simulink model "microchip_mcb_pmsm_foc_qep"  (R2021b)
settings: Solver=FixedStepDiscrete  StartTime=0.0  StopTime=8  FixedStep=Ts/2  RelTol=1e-3  EnableMultiTasking=on
InitFcn:
  | microchip_mcb_pmsm_foc_qep_data
values from neighbouring files (symbols this model uses):
  inverter = mcb_SetInverterParameters('Microchip_inverter')    [microchip_mcb_pmsm_foc_qep_data.m]
  PI_params = mcb.internal.SetControllerParameters(pmsm,inverter,PU_System,T_pwm,2*Ts,Ts_speed)    [microchip_mcb_pmsm_foc_qep_data.m]
  pmsm = mcb_SetPMSMMotorParameters('Microchip_motor')    [microchip_mcb_pmsm_foc_qep_data.m]
  PU_System = mcb_SetPUSystem(pmsm,inverter)    [microchip_mcb_pmsm_foc_qep_data.m]
  PWM_frequency = 20e3    (= 20000)    [microchip_mcb_pmsm_foc_qep_data.m]
  Ts = T_pwm    (= 5e-05)    [microchip_mcb_pmsm_foc_qep_data.m]
  Ts_motor = T_pwm/2    (= 2.5e-05)    [microchip_mcb_pmsm_foc_qep_data.m]
  Ts_simulink = T_pwm/2    (= 2.5e-05)    [microchip_mcb_pmsm_foc_qep_data.m]
  Ts_speed = 10*Ts    (= 0.0005)    [microchip_mcb_pmsm_foc_qep_data.m]
undefined symbols (not defined in the file or in its folder): A24, AD10, AD7, ADC0, LQFP144, MaxPer, ms, ns, PA0, PA1, PA10, PA11, PA12, PA13, PA18, PA9, PB0, PD18, PD19, PD24, PD25, PD26, Pin, Resol, SAME70Q21B, Unsigned, Vd_Ref_openLoop_PU
libraries: mcbcontrolslib x15, MCHP_Blockset x12, simulink x11, mcbpositiondecoderlib x4, mcbplantlib x1, autolibpmsmexterior x1
(part 3 of 4)

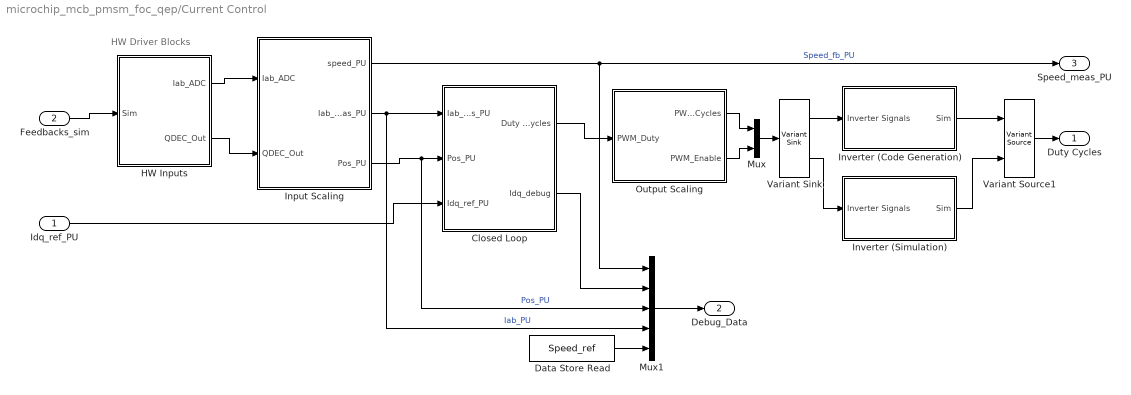
== system microchip_mcb_pmsm_foc_qep/Current Control ==
  note: HW Driver Blocks
  Idq_ref_PU : Inport
  Feedbacks_sim : Inport  Port=2
  Closed Loop : Subsystem
  Data Store Read : DataStoreRead  DataStoreName=Speed_ref  IndexOptions=Index vector (dialog)  Indices=1  OutputSizes=1
  HW Inputs : Subsystem  Variant=on  VariantControlMode=sim codegen switching
  Input Scaling : Subsystem
  Inverter (Code Generation) : Subsystem
  Inverter (Simulation) : Subsystem
  Mux : Mux  Inputs=2
  Mux1 : Mux  Inputs=5
  Output Scaling : Subsystem
  Variant Sink : VariantSink
  Variant Source1 : VariantSource
  Duty Cycles : Outport  InitialOutput=0  VectorParamsAs1DForOutWhenUnconnected=off
  Debug_Data : Outport  Port=2
  Speed_meas_PU : Outport  Port=3  InitialOutput=0  VectorParamsAs1DForOutWhenUnconnected=off
  wires:
  Closed Loop/1(Duty Cycles) -> Output Scaling/1(PWM_Duty)
  Output Scaling/2(PWM_Enable) -> Mux/2
  Input Scaling/1(speed_PU) -> Mux1/1, Speed_meas_PU/1  "Speed_fb_PU"
  Feedbacks_sim/1 -> HW Inputs/1(Sim)
  Input Scaling/2(Iab_meas_PU) -> Mux1/4, Closed Loop/1(Iab_meas_PU)  "Iab_PU"
  Input Scaling/3(Pos_PU) -> Mux1/3, Closed Loop/2(Pos_PU)  "Pos_PU"
  Variant Source1/1 -> Duty Cycles/1
  Output Scaling/1(PWM_Duty_Cycles) -> Mux/1
  Variant Sink/2 -> Inverter (Simulation)/1(Inverter Signals)
  Inverter (Code Generation)/1(Sim) -> Variant Source1/1
  Inverter (Simulation)/1(Sim) -> Variant Source1/2
  Variant Sink/1 -> Inverter (Code Generation)/1(Inverter Signals)
  Mux/1 -> Variant Sink/1
  HW Inputs/1(Iab_ADC) -> Input Scaling/1(Iab_ADC)
  HW Inputs/2(QDEC_Out) -> Input Scaling/2(QDEC_Out)
  Idq_ref_PU/1 -> Closed Loop/3(Idq_ref_PU)
  Mux1/1 -> Debug_Data/1
  Closed Loop/2(Idq_debug) -> Mux1/2
  Data Store Read/1 -> Mux1/5

== system microchip_mcb_pmsm_foc_qep/Heartbeat LED ==
  note: Heartbeat LED 1HZ
  Code generation : Subsystem
  RED_LED : Constant  OutDataTypeStr=uint16  SampleTime=0.25
  Simulation : Subsystem
  Variant Sink : VariantSink
  wires:
  RED_LED/1 -> Variant Sink/1
  Variant Sink/1 -> Code generation/1(In1)
  Variant Sink/2 -> Simulation/1(In1)

== system microchip_mcb_pmsm_foc_qep/Inverter and Motor - Plant Model ==
  Duty_Cycles : Inport
  Plant Model : Subsystem  Variant=on  VariantControlMode=sim codegen switching  VariantControl=Variant1  PropagateVariantConditions=on
  Feedbacks_sim : Outport  VectorParamsAs1DForOutWhenUnconnected=off
  wires:
  Duty_Cycles/1 -> Plant Model/1(Duty_Cycles)
  Plant Model/1(Feedbacks_sim) -> Feedbacks_sim/1

== system microchip_mcb_pmsm_foc_qep/Serial Receive ==
  CodeGen : Subsystem
  Data Store Write : DataStoreWrite  DataStoreName=Enable  IndexOptions=Index vector (dialog)  Indices=1  OutputSizes=1
  Sim : Subsystem
  Variant Source : VariantSource  VariantControlMode=sim codegen switching
  Variant Source1 : VariantSource  VariantControlMode=sim codegen switching
  SpeedRef : Outport
  wires:
  Variant Source/1 -> SpeedRef/1
  Variant Source1/1 -> Data Store Write/1
  Sim/1(SpeedRef) -> Variant Source/2
  Sim/2(Enable) -> Variant Source1/2
  CodeGen/1(SpeedRef) -> Variant Source/1
  CodeGen/2(Enable) -> Variant Source1/1

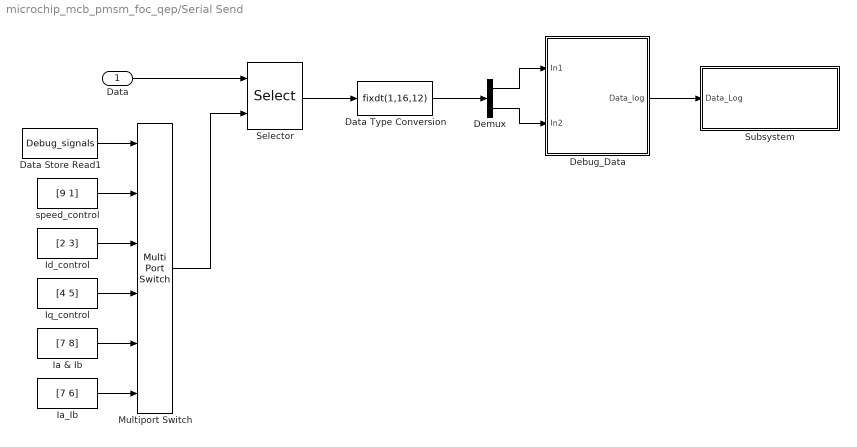
== system microchip_mcb_pmsm_foc_qep/Serial Send ==
  Data : Inport
  Data Store Read1 : DataStoreRead  DataStoreName=Debug_signals  IndexOptions=Index vector (dialog)  Indices=1  OutputSizes=1
  Data Type Conversion : DataTypeConversion  OutDataTypeStr=fixdt(1,16,12)  RndMeth=Simplest
  Debug_Data : Subsystem
  Demux : Demux  Outputs=2
  Ia & Ib : Constant  Value=[7 8]  OutDataTypeStr=uint16  SampleTime=-1
  Ia_Ib : Constant  Value=[7 6]  OutDataTypeStr=uint16  SampleTime=-1
  Id_control : Constant  Value=[2 3]  OutDataTypeStr=uint16  SampleTime=-1
  Iq_control : Constant  Value=[4 5]  OutDataTypeStr=uint16  SampleTime=-1
  Multiport Switch : MultiPortSwitch  Inputs=5  DiagnosticForDefault=Warning  OutDataTypeStr=uint16  RndMeth=Simplest
  Selector : Selector  InputPortWidth=9  IndexOptions=Index vector (port)  Indices=[1 3]  OutputSizes=1
  Subsystem : Subsystem
  speed_control : Constant  Value=[9 1]  OutDataTypeStr=uint16  SampleTime=-1
  wires:
  Debug_Data/1(Data_log) -> Subsystem/1(Data_Log)
  Demux/1 -> Debug_Data/1(In1)
  Demux/2 -> Debug_Data/2(In2)
  Data Type Conversion/1 -> Demux/1
  Selector/1 -> Data Type Conversion/1
  Data/1 -> Selector/1
  Data Store Read1/1 -> Multiport Switch/1
  Multiport Switch/1 -> Selector/2
  Ia_Ib/1 -> Multiport Switch/6
  Ia & Ib/1 -> Multiport Switch/5
  Iq_control/1 -> Multiport Switch/4
  Id_control/1 -> Multiport Switch/3
  speed_control/1 -> Multiport Switch/2

== system microchip_mcb_pmsm_foc_qep/Speed Control ==
  In1 : Inport
  Speed_Meas_PU : Inport  Port=2
  Data Store Write3 : DataStoreWrite  DataStoreName=Speed_ref  IndexOptions=Index vector (dialog)  Indices=1  OutputSizes=1
  Id_Ref : Constant  Value=0  OutDataTypeStr=dataType
  Mux : Mux  Inputs=2
  PI_Controller_Speed : Subsystem
  Speed_Ref_Selector : Subsystem
  IdqRef_PU : Outport  VectorParamsAs1DForOutWhenUnconnected=off
  wires:
  PI_Controller_Speed/1(Iq_ref) -> Mux/2
  Speed_Meas_PU/1 -> PI_Controller_Speed/2(N_fb)  "Speed_fb"
  Id_Ref/1 -> Mux/1
  Mux/1 -> IdqRef_PU/1
  Speed_Ref_Selector/1(Speed_Ref1) -> PI_Controller_Speed/1(N_ref)  "Speed_ref"
  In1/1 -> Data Store Write3/1, Speed_Ref_Selector/1(Speed_Ref)

== system microchip_mcb_pmsm_foc_qep/Current Control/Closed Loop ==
  Iab_meas_PU : Inport
  Pos_PU : Inport  Port=2
  Idq_ref_PU : Inport  Port=3
  Data Store Read1 : DataStoreRead  DataStoreName=EnClosedLoop  IndexOptions=Index vector (dialog)  Indices=1  OutputSizes=1
  Merge : Merge
  NOT : Logic  Operator=NOT  IconShape=distinctive  AllPortsSameDT=off  OutDataTypeStr=boolean
  OpenLoop : Subsystem
  Subsystem : Subsystem
  Duty Cycles : Outport  VectorParamsAs1DForOutWhenUnconnected=off
  Idq_debug : Outport  Port=2  VectorParamsAs1DForOutWhenUnconnected=off
  wires:
  Iab_meas_PU/1 -> Subsystem/1(Iab_meas_PU)  "Ia_Ib"
  Pos_PU/1 -> Subsystem/2(Pos_PU)
  Idq_ref_PU/1 -> Subsystem/3(Idq_ref_PU)
  Subsystem/1(Idq_debug) -> Idq_debug/1
  Merge/1 -> Duty Cycles/1
  OpenLoop/1(Duty Cycles) -> Merge/2
  Subsystem/2(Duty Cycles) -> Merge/1
  Data Store Read1/1 -> NOT/1, Subsystem/Enable
  NOT/1 -> OpenLoop/Enable

== system microchip_mcb_pmsm_foc_qep/Current Control/HW Inputs ==
  Sim : Inport
  Sensor Driver Blocks (codegen) : Subsystem  VariantControl=(codegen)
  Sensor Driver Blocks (sim) : Subsystem  VariantControl=(sim)
  Iab_ADC : Outport
  QDEC_Out : Outport  Port=2

== system microchip_mcb_pmsm_foc_qep/Current Control/Input Scaling ==
  Iab_ADC : Inport
  QDEC_Out : Inport  Port=2
  Calculate Phase Currents : Subsystem
  Calculate Position and Speed : Subsystem
  speed_PU : Outport
  Iab_meas_PU : Outport  Port=2
  Pos_PU : Outport  Port=3
  wires:
  Calculate Phase Currents/1(Iab_meas_PU) -> Iab_meas_PU/1
  Iab_ADC/1 -> Calculate Phase Currents/1(Iab_ADC)
  QDEC_Out/1 -> Calculate Position and Speed/1(Count)
  Calculate Position and Speed/1(Out1) -> speed_PU/1
  Calculate Position and Speed/2(ϴe) -> Pos_PU/1

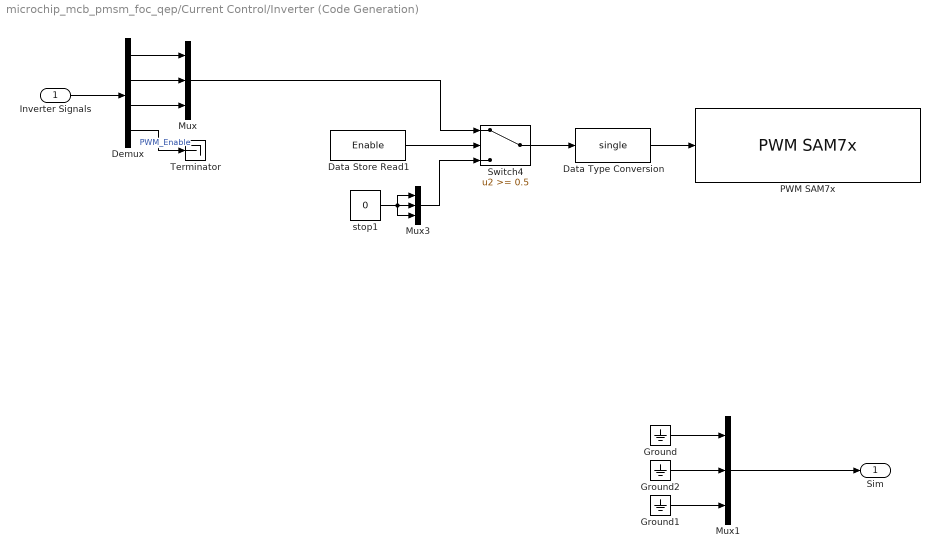
== system microchip_mcb_pmsm_foc_qep/Current Control/Inverter (Code Generation) ==
  Inverter Signals : Inport
  Data Store Read1 : DataStoreRead  DataStoreName=Enable  IndexOptions=Index vector (dialog)  Indices=1  OutputSizes=1
  Data Type Conversion : DataTypeConversion  OutDataTypeStr=single
  Demux : Demux
  Ground : Ground
  Ground1 : Ground
  Ground2 : Ground
  Mux : Mux  Inputs=3
  Mux1 : Mux  Inputs=3
  Mux3 : Mux  Inputs=3
  PWM SAM7x : MCHP_Blockset/PWM IO/PWM SAM7x  Priority=-2000  PWMx=PWM Controller 0  MaxPeriod_s=50e-6  PWM0_pinH0=Dynamic Options  PWM0_pinH0_TXT=PA11 / Pin[64]  PWM0_pinL0=Dynamic Options  PWM0_pinL0_TXT=PD24 / Pin[55]  PWM0_pinH1=Dynamic Options  PWM0_pinH1_TXT=PA12 / Pin[68]  PWM0_pinL1=Dynamic Options  PWM0_pinL1_TXT=PD25 / Pin[52]  PWM0_pinH2=Dynamic Options  PWM0_pinH2_TXT=PA13 / Pin[42]  PWM0_pinL2=Dynamic Options  PWM0_pinL2_TXT=PD26 / Pin[53]  PWM0_pinH3=Dynamic Options  PWM0_pinH3_TXT=Not Used  PWM0_pinL3=Dynamic Options  PWM0_pinL3_TXT=Not Used  PWM1_pinH0=Dynamic Options  PWM1_pinH0_TXT=Not Used  PWM1_pinL0=Dynamic Options  PWM1_pinL0_TXT=Not Used  PWM1_pinH1=Dynamic Options  PWM1_pinH1_TXT=Not Used  PWM1_pinL1=Dynamic Options  PWM1_pinL1_TXT=Not Used  PWM1_pinH2=Dynamic Options  PWM1_pinH2_TXT=Not Used  PWM1_pinL2=Dynamic Options  PWM1_pinL2_TXT=Not Used  PWM1_pinH3=Dynamic Options  PWM1_pinH3_TXT=Not Used  PWM1_pinL3=Dynamic Options  PWM1_pinL3_TXT=Not Used  PWM_Centered=on  PWM_SyncWithPWM0=on  PushPull_Mode=off  SampleTime=Ts  S_INPUT=[-1]  S_INPUT_Size=[3]  S_OUTPUT=[]  S_OUTPUT_Size=[]  S_ListCustomDatatype=S.S_ListCustomDatatype={};  evalin_ws=PWM0max0=MCHP_Fun.Hex2num('40AD4C0000000000');PWM1max0=MCHP_Fun.Hex2num('40AD4C0000000000');PWM2max0=MCHP_Fun.Hex2num('40AD4C0000000000');  MCHP_PWMC_CLOCK_REQUEST=''  MCHP_PWMC_CLOCK_RESULT=''  MCHP_USER_INTERRUPTS=0  MCHP_PORT={PWM0H0 }{PWMH0}4:1:P11;{PWM0L0 }{PWML0}4:1:P120;{PWM0H1 }{PWMH1}4:1:P12;{PWM0L1 }{PWML1}4:1:P121;{PWM0H2 }{PWMH2}4:1:P13;{PWM0L2 }{PWML2}4:1:P122;  MCHP_MASTERLINK=microchip_mcb_pmsm_foc_qep/Configurations/Microchip Master  invert_PWMH0=off  invert_PWML0=off  invert_PWMH1=off  invert_PWML1=off  invert_PWMH2=off  invert_PWML2=off  invert_PWMH3=off  invert_PWML3=off  InitPeriod_s=50e-6  InitDutyCycle_s=0  InitDeadTimeH_s=1e-6  InitDeadTimeL_s=1e-6  InitEventLine0_ComparatorValue_s=1e-7  InitEventLine1_ComparatorValue_s=[]  BlockInput_VectorScalar=Vectors (grouped by function)  BlockInput_Period=Not a block input  BlockInput_DutyCycle=a Floating Point input within range [-1 1]  BlockInput_DeadTime=Not a block input  BlockInput_OutputOverride=Not a block input  Fault_FPV0=Not forced  Fault_FPV1=Not forced  Fault_FPV2=Not forced  Fault_FPV3=Not forced  Fault_Input0=does nothing  Fault_Input0_FFIL=off  Fault_Input1=does nothing  Fault_Input1_FFIL=off  Fault_Input2=does nothing  Fault_Input2_FFIL=on  Fault_Input3=does nothing  Fault_Input3_FFIL=off  Fault_Input4=does nothing  Fault_Input4_FFIL=on  Fault_Input5=does nothing  Fault_Input5_FFIL=on  Fault_Input6=does nothing  Fault_Input6_FFIL=on  Fault_Input7=does nothing  Fault_Input7_FFIL=on
      settings: SourceProductName=MPLAB Device Blocks for Simulink
  Switch4 : Switch  Threshold=0.5  RndMeth=Simplest
  Terminator : Terminator
  stop1 : Constant  Value=0  OutDataTypeStr=dataType
  Sim : Outport  VectorParamsAs1DForOutWhenUnconnected=off
  wires:
  Inverter Signals/1 -> Demux/1
  Ground/1 -> Mux1/1
  Ground1/1 -> Mux1/3
  Ground2/1 -> Mux1/2
  Mux1/1 -> Sim/1
  Demux/1 -> Mux/1
  Demux/2 -> Mux/2
  Demux/3 -> Mux/3
  Switch4/1 -> Data Type Conversion/1
  Data Store Read1/1 -> Switch4/2
  Data Type Conversion/1 -> PWM SAM7x/1
  stop1/1 -> Mux3/3, Mux3/2, Mux3/1
  Mux/1 -> Switch4/1
  Mux3/1 -> Switch4/3
  Demux/4 -> Terminator/1  "PWM_Enable"

== system microchip_mcb_pmsm_foc_qep/Current Control/Inverter (Simulation) ==
  Inverter Signals : Inport
  Data Type Duplicate : DataTypeDuplicate
  Demux : Demux
  Mux : Mux  Inputs=3
  Mux2 : Mux  Inputs=3
  Subsystem : Subsystem
  Switch1 : Switch  Threshold=0.5  RndMeth=Simplest
  stop : Constant  Value=0  OutDataTypeStr=Inherit: Inherit via back propagation
  Sim : Outport  VectorParamsAs1DForOutWhenUnconnected=off
  wires:
  stop/1 -> Data Type Duplicate/2, Mux2/1, Mux2/3, Mux2/2
  Mux2/1 -> Switch1/3
  Switch1/1 -> Sim/1
  Inverter Signals/1 -> Demux/1
  Demux/4 -> Switch1/2  "PWM Enable"
  Mux/1 -> Subsystem/1(In1), Data Type Duplicate/1  "PWM Duty Cycles"
  Demux/1 -> Mux/1
  Demux/2 -> Mux/2
  Demux/3 -> Mux/3
  Subsystem/1(PWM_Duty_Cycles) -> Switch1/1  "test"

== system microchip_mcb_pmsm_foc_qep/Current Control/Output Scaling ==
  PWM_Duty : Inport
  Data Type Conversion : DataTypeConversion  OutDataTypeStr=dataType
  Enable : DataStoreRead  DataStoreName=Enable  IndexOptions=Index vector (dialog)  Indices=1  OutputSizes=1
  PWM_Duty_Cycles : Outport
  PWM_Enable : Outport  Port=2
  wires:
  Data Type Conversion/1 -> PWM_Enable/1
  Enable/1 -> Data Type Conversion/1
  PWM_Duty/1 -> PWM_Duty_Cycles/1

== system microchip_mcb_pmsm_foc_qep/Heartbeat LED/Code generation ==
  In1 : Inport
  DBG LED 1 : MCHP_Blockset/Digital IO/Digital Output Write  PORT=Dynamic Options  PORT_TXT="C   [ 0 : 31 ]"  PIN=23  PACK=off  SIMULTANEOUS=off  ORDERING=None  SampleTime=-1  MCHP_PORT={Digital Out}{DOU}1:1:C23;  MCHP_MASTERLINK=microchip_mcb_pmsm_foc_qep/Configurations/Microchip Master
      settings: SourceProductName=MPLAB Device Blocks for Simulink
  Delay 10Hz : Delay  DelayLength=1  InitialCondition=0  SampleTime=0.25
  Logical Operator : Logic  Operator=NOT  AllPortsSameDT=off  OutDataTypeStr=boolean
  Terminator : Terminator
  wires:
  Logical Operator/1 -> DBG LED 1/1, Delay 10Hz/1
  Delay 10Hz/1 -> Logical Operator/1
  In1/1 -> Terminator/1

== system microchip_mcb_pmsm_foc_qep/Heartbeat LED/Simulation ==
  In1 : Inport
  Simulation_Terminator : Terminator
  wires:
  In1/1 -> Simulation_Terminator/1

== system microchip_mcb_pmsm_foc_qep/Inverter and Motor - Plant Model/Plant Model ==
  Duty_Cycles : Inport
  Inverter and Motor (codegen) : Subsystem  VariantControl=(codegen)
  Inverter and Motor (sim) : Subsystem  VariantControl=(sim)
  Feedbacks_sim : Outport  VectorParamsAs1DForOutWhenUnconnected=off

== system microchip_mcb_pmsm_foc_qep/Serial Receive/CodeGen ==
  Data Store Write1 : DataStoreWrite  DataStoreName=Debug_signals  IndexOptions=Index vector (dialog)  Indices=1  OutputSizes=1
  Data Type Conversion : DataTypeConversion  OutDataTypeStr=uint16
  Subsystem : Subsystem
  Subsystem1 : Subsystem
  UART Rx : MCHP_Blockset/BUS UART/UART Rx  UART_REF=UART 0  Flag_Out=on  Rx_Size_popup=User defined  Rx_Size=1  S_Rx_Size=1  Split=Read all received char  SplitChar=10  OutputDefault_popup=do nothing (end of output vector will be undefined)  OutputDefault=-2  ORDERING=None  SampleTime=.001  MCHP_MASTERLINK=microchip_mcb_pmsm_foc_qep/Configurations/Microchip Master  MCHP_COMPILED_INFO="CompiledSampleTime= [0.0010000000000000000208   0 ];CompiledInportDataTypes=[    ];CompiledInportDataWidth=[];"
      settings: SourceProductName=MPLAB Device Blocks for Simulink
  SpeedRef : Outport
  Enable : Outport  Port=2
  wires:
  UART Rx/1 -> Data Type Conversion/1
  Subsystem/3(Debug Signal Selection) -> Data Store Write1/1
  UART Rx/2 -> Subsystem1/1(In1)
  Subsystem/2(Enable) -> Enable/1
  Subsystem/1(SpeedRef) -> SpeedRef/1
  Subsystem1/2(Data out) -> Subsystem/1(In1)
  Subsystem1/1(NewData) -> Subsystem/Enable
  Data Type Conversion/1 -> Subsystem1/Enable

== system microchip_mcb_pmsm_foc_qep/Serial Receive/Sim ==
  Data Type Conversion1 : DataTypeConversion  OutDataTypeStr=dataType  RndMeth=Simplest
  Data Type Conversion2 : DataTypeConversion  OutDataTypeStr=boolean  RndMeth=Simplest
  Step : Step  Time=5  Before=0.5  After=-0.5  OutDataTypeStr=single  SampleTime=0.001
  Step1 : Step  OutDataTypeStr=single  SampleTime=0.001
  SpeedRef : Outport
  Enable : Outport  Port=2
  wires:
  Step/1 -> Data Type Conversion1/1
  Data Type Conversion1/1 -> SpeedRef/1
  Step1/1 -> Data Type Conversion2/1
  Data Type Conversion2/1 -> Enable/1

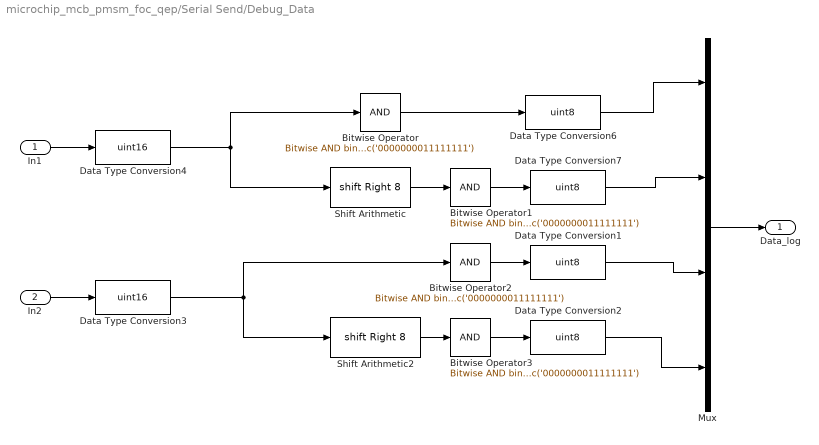
== system microchip_mcb_pmsm_foc_qep/Serial Send/Debug_Data ==
  In1 : Inport
  In2 : Inport  Port=2
  Bitwise Operator{,1..3} (4 alike) : simulink/Logic and Bit Operations/Bitwise Operator  logicop=AND  UseBitMask=on  BitMask=bin2dec('0000000011111111')  BitMaskRealWorld=Stored Integer
  Data Type Conversion{1..2,6..7} (4 alike) : DataTypeConversion  OutDataTypeStr=uint8  RndMeth=Simplest
  Data Type Conversion3 : DataTypeConversion  OutDataTypeStr=uint16  ConvertRealWorld=Stored Integer (SI)  RndMeth=Simplest
  Data Type Conversion4 : DataTypeConversion  OutDataTypeStr=uint16  ConvertRealWorld=Stored Integer (SI)  RndMeth=Simplest
  Mux : Mux
  Shift Arithmetic : ArithShift  BitShiftNumber=8  BitShiftDirection=Right
  Shift Arithmetic2 : ArithShift  BitShiftNumber=8  BitShiftDirection=Right
  Data_log : Outport
  wires:
  Data Type Conversion3/1 -> Bitwise Operator2/1, Shift Arithmetic2/1
  Bitwise Operator3/1 -> Data Type Conversion2/1
  Shift Arithmetic2/1 -> Bitwise Operator3/1
  Bitwise Operator1/1 -> Data Type Conversion7/1
  Data Type Conversion2/1 -> Mux/4
  Shift Arithmetic/1 -> Bitwise Operator1/1
  Bitwise Operator/1 -> Data Type Conversion6/1
  Data Type Conversion1/1 -> Mux/3
  Bitwise Operator2/1 -> Data Type Conversion1/1
  Data Type Conversion7/1 -> Mux/2
  Data Type Conversion6/1 -> Mux/1
  Data Type Conversion4/1 -> Shift Arithmetic/1, Bitwise Operator/1
  In1/1 -> Data Type Conversion4/1
  In2/1 -> Data Type Conversion3/1
  Mux/1 -> Data_log/1

== system microchip_mcb_pmsm_foc_qep/Serial Send/Subsystem ==
  note: Fast Serial Data Monitoring (32-bit)
  Data_Log : Inport
  Counter Limited : simulink/Sources/Counter Limited  uplimit=119  tsamp=-1
  Data : Subsystem  TreatAsAtomicUnit=on
  End : Subsystem  TreatAsAtomicUnit=on
  If : If  IfExpression=u1 == 0  ElseIfExpressions=u1 == 119
  Start : Subsystem  TreatAsAtomicUnit=on
  wires:
  If/3 -> Data/Action
  Counter Limited/1 -> If/1
  If/2 -> End/Action
  If/1 -> Start/Action
  Data_Log/1 -> End/1(Data), Start/1(Data), Data/1(Data)

== system microchip_mcb_pmsm_foc_qep/Speed Control/PI_Controller_Speed ==
  N_ref : Inport
  N_fb : Inport  Port=2
  AND : Logic  IconShape=distinctive  AllPortsSameDT=off  OutDataTypeStr=boolean
  Data Store Read2 : DataStoreRead  DataStoreName=EnClosedLoop  IndexOptions=Index vector (dialog)  Indices=1  OutputSizes=1
  Data Store Read1 : DataStoreRead  DataStoreName=Enable  IndexOptions=Index vector (dialog)  Indices=1  OutputSizes=1
  Discrete PI Controller with anti-windup & reset : mcbcontrolslib/Discrete PI Controller  with anti-windup & reset  UpperSaturationLimit=0.5  LowerSaturationLimit=-0.5
      settings: SourceProductBaseCode=MT
  Ki1 : Constant  Value=PI_params.Ki_speed*Ts_speed  OutDataTypeStr=dataType  SampleTime=-1
  Ki2 : Constant  Value=0  OutDataTypeStr=dataType  SampleTime=-1
  Kp1 : Constant  Value=PI_params.Kp_speed  OutDataTypeStr=dataType  SampleTime=-1
  Logical Operator : Logic  Operator=NOT  IconShape=distinctive  AllPortsSameDT=off  OutDataTypeStr=boolean
  Sum : Sum  Inputs=|+-  OutDataTypeStr=Inherit: Same as first input
  Iq_ref : Outport  VectorParamsAs1DForOutWhenUnconnected=off
  wires:
  Discrete PI Controller with anti-windup & reset/1 -> Iq_ref/1
  Ki1/1 -> Discrete PI Controller with anti-windup & reset/3
  Kp1/1 -> Discrete PI Controller with anti-windup & reset/2
  N_fb/1 -> Sum/2
  N_ref/1 -> Sum/1
  Sum/1 -> Discrete PI Controller with anti-windup & reset/1
  Logical Operator/1 -> Discrete PI Controller with anti-windup & reset/4
  Ki2/1 -> Discrete PI Controller with anti-windup & reset/5
  Data Store Read1/1 -> AND/1
  Data Store Read2/1 -> AND/2
  AND/1 -> Logical Operator/1

== system microchip_mcb_pmsm_foc_qep/Speed Control/Speed_Ref_Selector ==
  Speed_Ref : Inport
  Constant : Constant  Value=0  OutDataTypeStr=dataType
  Constant1 : Constant  Value=-0.1  OutDataTypeStr=dataType
  Data Store Read : DataStoreRead  DataStoreName=Speed_ref  IndexOptions=Index vector (dialog)  Indices=1  OutputSizes=1
  Data Store Read1 : DataStoreRead  DataStoreName=EnClosedLoop  IndexOptions=Index vector (dialog)  Indices=1  OutputSizes=1
  IIR Filter : mcbcontrolslib/IIR Filter  VariantControl=Low Pass Filter  VariantSelect=Low-pass  Filter_constant=0.001*(Ts_speed/Ts)  advancedSettings=off  Ts=50e-6  cutOff_freq=32.1525
      settings: SourceProductBaseCode=MT
  Switch : Switch  Criteria=u2 > Threshold
  Switch1 : Switch  Criteria=u2 > Threshold
  Speed_Ref1 : Outport
  wires:
  IIR Filter/1 -> Speed_Ref1/1  "Speed_Ref"
  Data Store Read1/1 -> Switch/2
  Switch/1 -> IIR Filter/1  "Speed_Ref"
  Constant/1 -> Switch1/1
  Data Store Read/1 -> Switch1/2
  Switch1/1 -> Switch/3
  Speed_Ref/1 -> Switch/1
  Constant1/1 -> Switch1/3

== system microchip_mcb_pmsm_foc_qep/Current Control/Closed Loop/OpenLoop ==
  Enable : EnablePort
  Constant : Constant  Value=0.15  OutDataTypeStr=dataType
  Constant1 : Constant  Value=0  OutDataTypeStr=dataType
  Enable1 : DataStoreRead  DataStoreName=Enable  IndexOptions=Index vector (dialog)  Indices=1  OutputSizes=1
  Inverse Park Transform : mcbcontrolslib/Inverse Park Transform  AxisAlignment=D-axis
  Mode Selector : Subsystem
  Mux1 : Mux  Inputs=3
  Sine-Cosine Lookup : mcbcontrolslib/Sine-Cosine Lookup  AngleInput=Per-unit  N_points=1024
      settings: SourceProductBaseCode=MT
  Space Vector Generator : mcbcontrolslib/PWM Reference Generator  inSignal=Valphabeta  modType=SVM: space vector modulation
      settings: SourceProductBaseCode=MT
  Duty Cycles : Outport  VectorParamsAs1DForOutWhenUnconnected=off
  wires:
  Mode Selector/1(PositionOffsetEn) -> Sine-Cosine Lookup/1  "Pos_open"
  Constant1/1 -> Inverse Park Transform/2
  Constant/1 -> Inverse Park Transform/1
  Space Vector Generator/3 -> Mux1/3
  Sine-Cosine Lookup/2 -> Inverse Park Transform/4
  Space Vector Generator/1 -> Mux1/1
  Sine-Cosine Lookup/1 -> Inverse Park Transform/3
  Inverse Park Transform/2 -> Space Vector Generator/2
  Space Vector Generator/2 -> Mux1/2
  Inverse Park Transform/1 -> Space Vector Generator/1
  Mux1/1 -> Duty Cycles/1
  Enable1/1 -> Mode Selector/Enable

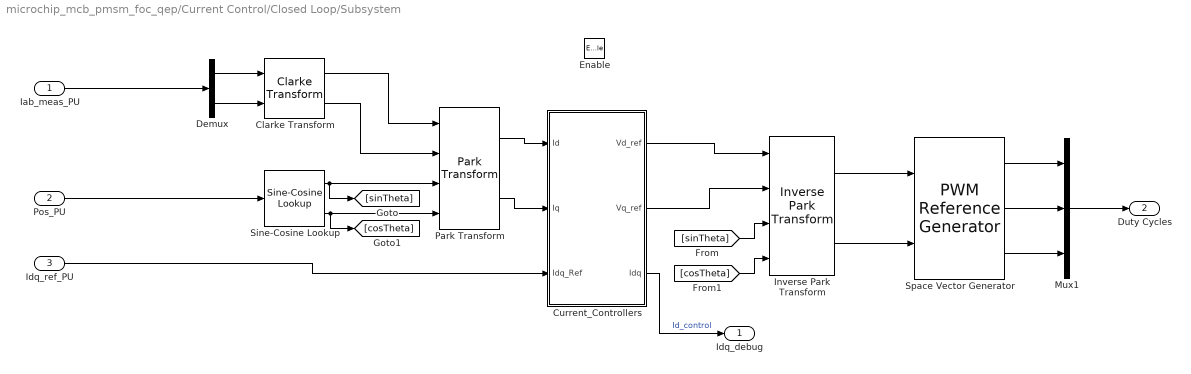
== system microchip_mcb_pmsm_foc_qep/Current Control/Closed Loop/Subsystem ==
  Iab_meas_PU : Inport
  Pos_PU : Inport  Port=2
  Idq_ref_PU : Inport  Port=3
  Enable : EnablePort
  Clarke Transform : mcbcontrolslib/Clarke Transform  VariantControl=Variant2
  Current_Controllers : Subsystem
  Demux : Demux  Outputs=2
  Inverse Park Transform : mcbcontrolslib/Inverse Park Transform  AxisAlignment=D-axis
  Mux1 : Mux  Inputs=3
  Park Transform : mcbcontrolslib/Park Transform  AxisAlignment=D-axis
      settings: SourceProductBaseCode=MT
  Sine-Cosine Lookup : mcbcontrolslib/Sine-Cosine Lookup  AngleInput=Per-unit  N_points=1024
      settings: SourceProductBaseCode=MT
  Space Vector Generator : mcbcontrolslib/PWM Reference Generator  inSignal=Valphabeta  modType=SVM: space vector modulation
      settings: SourceProductBaseCode=MT
  Idq_debug : Outport  VectorParamsAs1DForOutWhenUnconnected=off
  Duty Cycles : Outport  Port=2  VectorParamsAs1DForOutWhenUnconnected=off
  wires:
  Pos_PU/1 -> Sine-Cosine Lookup/1
  Inverse Park Transform/2 -> Space Vector Generator/2
  [cosTheta] -> Inverse Park Transform/4
  Inverse Park Transform/1 -> Space Vector Generator/1
  Sine-Cosine Lookup/1 -> [sinTheta], Park Transform/3
  Current_Controllers/1(Vd_ref) -> Inverse Park Transform/1
  Sine-Cosine Lookup/2 -> Park Transform/4, [cosTheta]
  Clarke Transform/2 -> Park Transform/2
  Clarke Transform/1 -> Park Transform/1
  Space Vector Generator/3 -> Mux1/3
  Space Vector Generator/1 -> Mux1/1
  Current_Controllers/3(Idq) -> Idq_debug/1  "Id_control"
  Mux1/1 -> Duty Cycles/1
  Space Vector Generator/2 -> Mux1/2
  Iab_meas_PU/1 -> Demux/1
  Demux/2 -> Clarke Transform/2
  [sinTheta] -> Inverse Park Transform/3
  Demux/1 -> Clarke Transform/1
  Park Transform/2 -> Current_Controllers/2(Iq)
  Current_Controllers/2(Vq_ref) -> Inverse Park Transform/2
  Idq_ref_PU/1 -> Current_Controllers/3(Idq_Ref)
  Park Transform/1 -> Current_Controllers/1(Id)

== system microchip_mcb_pmsm_foc_qep/Current Control/HW Inputs/Sensor Driver Blocks (codegen) ==
  Sim : Inport
  ADC SAMx1 : MCHP_Blockset/Analog IO/ADC SAMx7  Priority=-2000  AFECx=AFE Controller 0  SIGNMODE_SingleEnded=Unsigned (uint16)  SIGNMODE_Differential=Unsigned (uint16)  AFEC0_seq0=Dynamic Options  AFEC0_seq0_TXT="AD0 / PD30   &   AD6 / PA17"  AFEC1_seq0=Dynamic Options  AFEC1_seq0_TXT=Not used  AFEC0_seq1=Dynamic Options  AFEC0_seq1_TXT=AD7 / PA18  AFEC1_seq1=Dynamic Options  AFEC1_seq1_TXT=Not used  AFEC0_seq2=Dynamic Options  AFEC0_seq2_TXT=AD10 / PB0  AFEC1_seq2=Dynamic Options  AFEC1_seq2_TXT=Not used  AFEC0_seq3=Dynamic Options  AFEC0_seq3_TXT=Not used  AFEC1_seq3=Dynamic Options  AFEC1_seq3_TXT=Not used  AFEC0_seq4=Dynamic Options  AFEC0_seq4_TXT=Not used  AFEC1_seq4=Dynamic Options  AFEC1_seq4_TXT=Not used  AFEC0_seq5=Dynamic Options  AFEC0_seq5_TXT=Not used  AFEC1_seq5=Dynamic Options  AFEC1_seq5_TXT=Not used  AFEC0_seq6=Dynamic Options  AFEC0_seq6_TXT=Not used  AFEC1_seq6=Dynamic Options  AFEC1_seq6_TXT=Not used  AFEC0_seq7=Dynamic Options  AFEC0_seq7_TXT=Not used  AFEC1_seq7=Dynamic Options  AFEC1_seq7_TXT=Not used  AFEC0_seq8=Dynamic Options  AFEC0_seq8_TXT=Not used  AFEC1_seq8=Dynamic Options  AFEC1_seq8_TXT=Not used  AFEC0_seq9=Dynamic Options  AFEC0_seq9_TXT=Not used  AFEC1_seq9=Dynamic Options  AFEC1_seq9_TXT=Not used  AFEC0_seq10=Dynamic Options  AFEC0_seq10_TXT=Not used  AFEC1_seq10=Dynamic Options  AFEC1_seq10_TXT=Not used  AFEC0_seq11=Dynamic Options  AFEC0_seq11_TXT=Not used  AFEC1_seq11=Dynamic Options  AFEC1_seq11_TXT=Not used  SampleTime=Ts  S_INPUT=[-1]  S_INPUT_Size=[3]  S_OUTPUT=[]  S_OUTPUT_Size=[]  S_ListCustomDatatype=S.S_ListCustomDatatype={};  MCHP_AFECC_CLOCK_REQUEST=''  MCHP_AFECC_CLOCK_RESULT=''  MCHP_USER_INTERRUPTS=0  MCHP_PORT={AD0 AFEC0}{AD0}15:2:P126;{AD6 AFEC0}{AD6}15:2:P17;{AD7 AFEC0}{AD7}15:2:P18;{AD10 AFEC0}{AD10}15:2:P32;  MCHP_MASTERLINK=microchip_mcb_pmsm_foc_qep/Configurations/Microchip Master  Rin=< 200 Ohm  RES=12-bit Standard  AFEC0_Synchronisation=Triggered by user defined source  AFEC0_Trig=PWM0 event line 0  AFEC0_TrigTimeStep=on  AFEC1_Synchronisation=Triggered by user defined source  AFEC1_Trig=PWM1 event line 0  AFEC1_TrigTimeStep=off  ADC_TrigInfo=0  AFEC0_seq0_GAIN=1  AFEC1_seq0_GAIN=1  AFEC0_seq1_GAIN=1  AFEC1_seq1_GAIN=1  AFEC0_seq2_GAIN=1  AFEC1_seq2_GAIN=1  AFEC0_seq3_GAIN=1  AFEC1_seq3_GAIN=1  AFEC0_seq4_GAIN=1  AFEC1_seq4_GAIN=1  AFEC0_seq5_GAIN=1  AFEC1_seq5_GAIN=1  AFEC0_seq6_GAIN=1  AFEC1_seq6_GAIN=1  AFEC0_seq7_GAIN=1  AFEC1_seq7_GAIN=1  AFEC0_seq8_GAIN=1  AFEC1_seq8_GAIN=1  AFEC0_seq9_GAIN=1  AFEC1_seq9_GAIN=1  AFEC0_seq10_GAIN=1  AFEC1_seq10_GAIN=1  AFEC0_seq11_GAIN=1  AFEC1_seq11_GAIN=1  AFEC0_seq0_OFFSET=0  AFEC1_seq0_OFFSET=0  AFEC0_seq1_OFFSET=0  AFEC1_seq1_OFFSET=0  AFEC0_seq2_OFFSET=0  AFEC1_seq2_OFFSET=0  AFEC0_seq3_OFFSET=0  AFEC1_seq3_OFFSET=0  AFEC0_seq4_OFFSET=0  AFEC1_seq4_OFFSET=0  AFEC0_seq5_OFFSET=0  AFEC1_seq5_OFFSET=0  AFEC0_seq6_OFFSET=0  AFEC1_seq6_OFFSET=0  AFEC0_seq7_OFFSET=0  AFEC1_seq7_OFFSET=0  AFEC0_seq8_OFFSET=0  AFEC1_seq8_OFFSET=0  AFEC0_seq9_OFFSET=0  AFEC1_seq9_OFFSET=0  AFEC0_seq10_OFFSET=0  AFEC1_seq10_OFFSET=0  AFEC0_seq11_OFFSET=0  AFEC1_seq11_OFFSET=0
      settings: SourceProductName=MPLAB Device Blocks for Simulink
  Data Store Read : DataStoreRead  DataStoreName=EnPosOffset  IndexOptions=Index vector (dialog)  Indices=1  OutputSizes=1
  Mux : Mux  Inputs=2
  QDEC : MCHP_Blockset/QEI/QDEC  QDEC_REF=Dynamic Options  QDEC_REF_TXT=TC0  PHA_PIN=Dynamic Options  PHA_PIN_TXT=PA0 / Pin[102]  PHB_PIN=Dynamic Options  PHB_PIN_TXT=PA1 / Pin[99]  IDX_PIN=Dynamic Options  IDX_PIN_TXT=not used  INVERT_PHA=off  INVERT_PHB=off  INVERT_IDX=off  SWAP_PHA_PHB=off  SampleTime=Ts  MCHP_PORT={TC0}{TIOA0}3:0:P0;{TC0}{TIOB0}3:0:P1;  MCHP_MASTERLINK=microchip_mcb_pmsm_foc_qep/Configurations/Microchip Master  MCHP_TIMER_REQUEST={Quadrature Decoder (Phase Counter)}{QDEC0}20:4:4:0:[1]:65535;{Quadrature Decoder (IDX Counter)}{QDEC0}20:4:4:0:[2]:65535;{Quadrature Decoder (Speed Measurement Time Base)}{QDEC0}20:4:4:0:[3]:65535;  MCHP_TIMER_RESULT=[1 65535]  QDEC_MODE=Position  POSITION_OUTPUT=is a 16 bits unsigned block output  INDEX_OUTPUT=is not a block output  RESET_INPUT=on  POSITION_RESET_MODE=at user defined value  RESET_EDGE=rising edge  POSITION_RESET_VALUE=1000  SPEED_TIME_BASE=Dynamic Options  SPEED_TIME_BASE_TXT=Resol: 53.33(ns) - MaxPer: 3.5(ms)  SPEED_OUTPUT=is a 16 bits unsigned block output  DIR_OUTPUT=is not a block output  DIRCHG_OUTPUT=is not a block output  AUTO_CORRECTION=off  MAX_PERIOD_FILTER=Dynamic Options  MAX_PERIOD_FILTER_TXT=420(ns)  MAXCMP=disabled  MPE_OUTPUT=is not a block output  QERR_OUTPUT=is not a block output
      settings: SourceProductName=MPLAB Device Blocks for Simulink
  Terminator : Terminator
  Terminator1 : Terminator
  Terminator2 : Terminator
  Iab_ADC : Outport
  QDEC_Out : Outport  Port=2
  wires:
  Sim/1 -> Terminator/1
  Mux/1 -> Iab_ADC/1
  ADC SAMx1/4 -> Terminator2/1
  ADC SAMx1/3 -> Terminator1/1
  ADC SAMx1/1 -> Mux/1
  ADC SAMx1/2 -> Mux/2
  QDEC/1 -> QDEC_Out/1
  Data Store Read/1 -> QDEC/1

== system microchip_mcb_pmsm_foc_qep/Current Control/HW Inputs/Sensor Driver Blocks (sim) ==
  Sim : Inport
  Demux : Demux  Outputs=3
  Mux : Mux  Inputs=2
  Iab_ADC : Outport
  QDEC_Out : Outport  Port=2
  wires:
  Sim/1 -> Demux/1
  Demux/3 -> QDEC_Out/1
  Mux/1 -> Iab_ADC/1
  Demux/2 -> Mux/2
  Demux/1 -> Mux/1

== system microchip_mcb_pmsm_foc_qep/Current Control/Input Scaling/Calculate Phase Currents ==
  Iab_ADC : Inport
  Add : Sum  Inputs=-+
  Data Store Read : DataStoreRead  DataStoreName=IaOffset  IndexOptions=Index vector (dialog)  Indices=1  OutputSizes=1
  Data Store Read1 : DataStoreRead  DataStoreName=IbOffset  IndexOptions=Index vector (dialog)  Indices=1  OutputSizes=1
  Data Type Conversion : DataTypeConversion  OutDataTypeStr=int32  ConvertRealWorld=Stored Integer (SI)
  Data Type Conversion1 : DataTypeConversion  OutDataTypeStr=dataType
  Gain1 : Gain  Gain=1/2048  OutDataTypeStr=Inherit: Same as input  ParamDataTypeStr=Inherit: Same as input
  Mux1 : Mux  Inputs=2
  Unary Minus : UnaryMinus  Commented=through
  Iab_meas_PU : Outport  VectorParamsAs1DForOutWhenUnconnected=off
  wires:
  Mux1/1 -> Add/1
  Data Type Conversion/1 -> Add/2
  Add/1 -> Data Type Conversion1/1
  Iab_ADC/1 -> Data Type Conversion/1
  Data Store Read1/1 -> Mux1/2
  Data Store Read/1 -> Mux1/1
  Unary Minus/1 -> Iab_meas_PU/1
  Data Type Conversion1/1 -> Gain1/1
  Gain1/1 -> Unary Minus/1

== system microchip_mcb_pmsm_foc_qep/Current Control/Input Scaling/Calculate Position and Speed ==
  Count : Inport
  Data Store Read : DataStoreRead  DataStoreName=EnPosOffset  IndexOptions=Index vector (dialog)  Indices=1  OutputSizes=1
  IIR Filter : mcbcontrolslib/IIR Filter  VariantControl=Low Pass Filter  VariantSelect=Low-pass  Filter_constant=0.1  advancedSettings=off  Ts=50e-6  cutOff_freq=353.6777
      settings: SourceProductBaseCode=MT
  Mechanical to Electrical Position : mcbpositiondecoderlib/Mechanical to Electrical Position  NrPP=pmsm.p  selectedRange=Per unit  MechOfstInputType=Input port  mechOffsetIn=0  maxAngleIn=1  InputDataType=dataType  VariantSelect=floating-point
      settings: SourceProductBaseCode=MT
  Position Offset : Subsystem
  Position Offset Sim : Constant  Value=0  OutDataTypeStr=Inherit: Inherit via back propagation
  Quadrature Decoder : mcbpositiondecoderlib/Quadrature Decoder  EncoderSlitsPerRevolution=pmsm.QEPSlits  EncoderCountsPerSlit=4  CounterSize=16 bits  ExternalIndexCount=off  PositionUnit=Per unit  PositionDataType=dataType
      settings: SourceProductBaseCode=MT
  Speed Measurement : mcbpositiondecoderlib/Speed Measurement  PositionUnit=Per unit  PositionScalingDatatype=uint32  SpeedCalculationMode=Time interval for speed calculation  SampleTimeAsync=Ts  MaximumApplicationSpeed=1000  SpeedResolution=5e-6  DelayLength=20  MaximumMeasurableSpeed=29999  MeasurableSpeedResolution=1.397e-05  SpeedUnit=Per unit based on dialog  PerUnitSpeed=PU_System.N_base  SpeedDataType=dataType
      settings: SourceProductBaseCode=MT
  Variant Source2 : VariantSource  VariantControlMode=sim codegen switching
  Out1 : Outport
  ϴe : Outport  Port=2
  wires:
  Count/1 -> Quadrature Decoder/1
  Data Store Read/1 -> Position Offset/Enable
  Position Offset/1(Offset) -> Variant Source2/1
  Quadrature Decoder/1 -> Mechanical to Electrical Position/1, Position Offset/1(Iab), Speed Measurement/1  "Pos"
  Position Offset Sim/1 -> Variant Source2/2
  Speed Measurement/1 -> IIR Filter/1
  Variant Source2/1 -> Mechanical to Electrical Position/2
  Mechanical to Electrical Position/1 -> ϴe/1
  IIR Filter/1 -> Out1/1

== system microchip_mcb_pmsm_foc_qep/Current Control/Inverter (Simulation)/Subsystem ==
  In1 : Inport
  Constant : Constant  Value=0.5  OutDataTypeStr=dataType
  Gain : Gain  Gain=0.5  OutDataTypeStr=Inherit: Same as input
  Sum : Sum  Inputs=|++
  PWM_Duty_Cycles : Outport
  wires:
  Gain/1 -> Sum/1
  Constant/1 -> Sum/2
  In1/1 -> Gain/1
  Sum/1 -> PWM_Duty_Cycles/1  "PWM_Duty_Cycles"

== system microchip_mcb_pmsm_foc_qep/Inverter and Motor - Plant Model/Plant Model/Inverter and Motor (codegen) ==
  Duty_Cycles : Inport
  Ground : Ground
  Terminator : Terminator
  Feedbacks_sim : Outport  VectorParamsAs1DForOutWhenUnconnected=off
  wires:
  Duty_Cycles/1 -> Terminator/1
  Ground/1 -> Feedbacks_sim/1

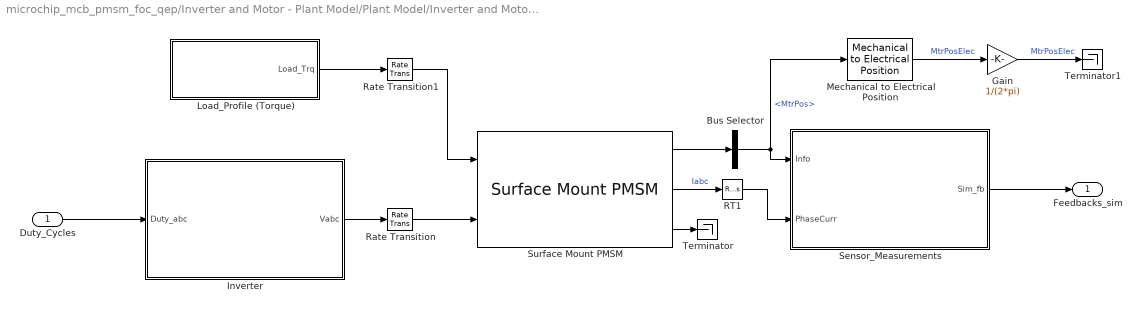
== system microchip_mcb_pmsm_foc_qep/Inverter and Motor - Plant Model/Plant Model/Inverter and Motor (sim) ==
  Duty_Cycles : Inport
  Bus Selector : BusSelector  OutputSignals=MtrPos
  Gain : Gain  Gain=1/(2*pi)  OutDataTypeStr=Inherit: Same as input
  Inverter : Subsystem
  Load_Profile (Torque) : Subsystem
  Mechanical to Electrical Position : mcbpositiondecoderlib/Mechanical to Electrical Position  NrPP=pmsm.p  selectedRange=Radians  MechOfstInputType=Specify via dialog  mechOffsetIn=0  maxAngleIn=2*pi  InputDataType=single  VariantSelect=floating-point
      settings: SourceProductBaseCode=MT
  RT1 : RateTransition  Deterministic=off  OutPortSampleTime=Ts_simulink
  Rate Transition : RateTransition  Deterministic=off  OutPortSampleTime=Ts_motor
  Rate Transition1 : RateTransition  Deterministic=off  OutPortSampleTime=Ts_motor
  Sensor_Measurements : Subsystem
  Surface Mount PMSM : autolibpmsmexterior/Surface Mount PMSM  port_config=Torque  sim_type=Discrete  Ts=Ts_motor  FilePath=surfacepmsm_motordata.m  P=pmsm.p  Rs=pmsm.Rs + inverter.R_board  Ldq_=pmsm.Ld  KConstText=Permanent flux linkage constant (lambda_pm):  lambda_pm=pmsm.FluxPM  Ke=159.9771  Kt=1.323  mechanical=[pmsm.J, pmsm.B, 0]  idq0=[0 0]  theta_init=0  omega_init=0  KConst=pmsm.FluxPM  lambda_pm_calc=pmsm.FluxPM  RefBlkName='autolibpmsmexterior/Surface Mount PMSM'  aMode=5  Ldq="[0.00078136  0.00078136]"
      settings: SourceProductBaseCode=PW,DR,MT,UV,VE
  Terminator : Terminator
  Terminator1 : Terminator
  Feedbacks_sim : Outport  VectorParamsAs1DForOutWhenUnconnected=off
  wires:
  Inverter/1(Vabc) -> Rate Transition/1
  Surface Mount PMSM/2 -> RT1/1  "Iabc"
  Sensor_Measurements/1(Sim_fb) -> Feedbacks_sim/1
  Surface Mount PMSM/3 -> Terminator/1
  Load_Profile (Torque)/1(Load_Trq) -> Rate Transition1/1
  Duty_Cycles/1 -> Inverter/1(Duty_abc)
  Rate Transition/1 -> Surface Mount PMSM/2
  Rate Transition1/1 -> Surface Mount PMSM/1
  RT1/1 -> Sensor_Measurements/2(PhaseCurr)
  Gain/1 -> Terminator1/1  "MtrPosElec"
  Mechanical to Electrical Position/1 -> Gain/1  "MtrPosElec"
  Bus Selector/1 -> Mechanical to Electrical Position/1, Sensor_Measurements/1(Info)  "<MtrPos>"
  Surface Mount PMSM/1 -> Bus Selector/1

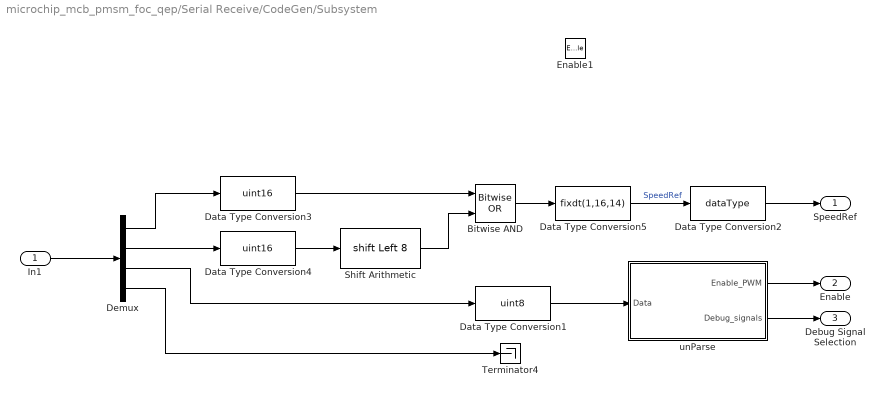
== system microchip_mcb_pmsm_foc_qep/Serial Receive/CodeGen/Subsystem ==
  In1 : Inport
  Enable1 : EnablePort
  Bitwise AND : simulink/Logic and Bit Operations/Bitwise Operator  logicop=OR  UseBitMask=off  NumInputPorts=2  BitMask=bin2dec('11011001')  BitMaskRealWorld=Stored Integer
  Data Type Conversion1 : DataTypeConversion  OutDataTypeStr=uint8  RndMeth=Simplest
  Data Type Conversion2 : DataTypeConversion  OutDataTypeStr=dataType  RndMeth=Simplest
  Data Type Conversion3 : DataTypeConversion  OutDataTypeStr=uint16  RndMeth=Simplest
  Data Type Conversion4 : DataTypeConversion  OutDataTypeStr=uint16  RndMeth=Simplest
  Data Type Conversion5 : DataTypeConversion  OutDataTypeStr=fixdt(1,16,14)  ConvertRealWorld=Stored Integer (SI)  RndMeth=Zero
  Demux : Demux
  Shift Arithmetic : ArithShift  BitShiftNumber=8  BitShiftDirection=Left
  Terminator4 : Terminator
  unParse : Subsystem
  SpeedRef : Outport
  Enable : Outport  Port=2
  Debug Signal Selection : Outport  Port=3
  wires:
  Data Type Conversion4/1 -> Shift Arithmetic/1
  Data Type Conversion3/1 -> Bitwise AND/1
  In1/1 -> Demux/1
  unParse/2(Debug_signals) -> Debug Signal Selection/1
  Data Type Conversion2/1 -> SpeedRef/1
  Demux/3 -> Data Type Conversion1/1
  Bitwise AND/1 -> Data Type Conversion5/1
  unParse/1(Enable_PWM) -> Enable/1
  Data Type Conversion1/1 -> unParse/1(Data)
  Demux/2 -> Data Type Conversion4/1
  Demux/4 -> Terminator4/1
  Shift Arithmetic/1 -> Bitwise AND/2
  Data Type Conversion5/1 -> Data Type Conversion2/1  "SpeedRef"
  Demux/1 -> Data Type Conversion3/1

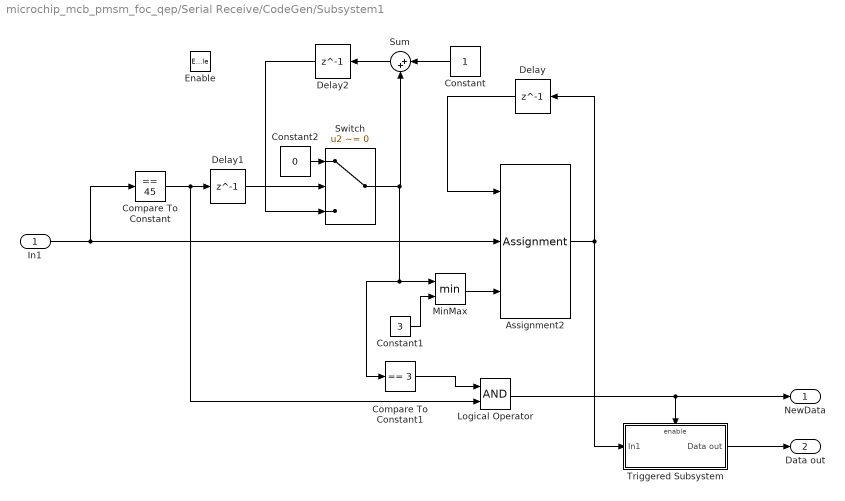
== system microchip_mcb_pmsm_foc_qep/Serial Receive/CodeGen/Subsystem1 ==
  In1 : Inport
  Enable : EnablePort
  Assignment2 : Assignment  IndexMode=Zero-based  DiagnosticForDimensions=Warning  IndexOptions=Starting index (port)  Indices=1  OutputSizes=1
  Compare To Constant : simulink/Logic and Bit Operations/Compare To Constant  relop===  const=45  OutDataTypeStr=boolean
  Compare To Constant1 : simulink/Logic and Bit Operations/Compare To Constant  relop===  const=3  OutDataTypeStr=boolean
  Constant : Constant  OutDataTypeStr=uint16  SampleTime=-1
  Constant1 : Constant  Value=3  OutDataTypeStr=uint16  SampleTime=-1
  Constant2 : Constant  Value=0  OutDataTypeStr=uint16  SampleTime=-1
  Delay : Delay  DelayLength=1  InitialCondition=[0 0 0 0]
  Delay1 : Delay  DelayLength=1  InitialCondition=0
  Delay2 : Delay  DelayLength=1  InitialCondition=0
  Logical Operator : Logic  AllPortsSameDT=off  OutDataTypeStr=boolean
  MinMax : MinMax  Inputs=2
  Sum : Sum  Inputs=|++
  Switch : Switch  Criteria=u2 ~= 0
  Triggered Subsystem : Subsystem  TreatAsAtomicUnit=on
  NewData : Outport  OutputWhenDisabled=reset  InitialOutput=0
  Data out : Outport  Port=2
  wires:
  Logical Operator/1 -> Triggered Subsystem/Enable, NewData/1
  Triggered Subsystem/1(Data out) -> Data out/1
  Constant2/1 -> Switch/1
  Delay1/1 -> Switch/2
  Switch/1 -> MinMax/1, Compare To Constant1/1, Sum/2
  Sum/1 -> Delay2/1
  MinMax/1 -> Assignment2/3
  Constant1/1 -> MinMax/2
  Constant/1 -> Sum/1
  In1/1 -> Assignment2/2, Compare To Constant/1
  Compare To Constant1/1 -> Logical Operator/1
  Compare To Constant/1 -> Delay1/1, Logical Operator/2
  Delay2/1 -> Switch/3
  Delay/1 -> Assignment2/1
  Assignment2/1 -> Delay/1, Triggered Subsystem/1(In1)

== system microchip_mcb_pmsm_foc_qep/Serial Send/Subsystem/Data ==
  Data : Inport
  Action Port : ActionPort  ActionPortLabel=else
  UART Tx : MCHP_Blockset/BUS UART/UART Tx  UART_REF=UART 0  ORDERING=None  AllOrNothing=off  SampleTime=-1  MCHP_MASTERLINK=microchip_mcb_pmsm_foc_qep/Configurations/Microchip Master  NSend_Input=off  UART_String=off  NSend_Output=off
      settings: SourceProductName=MPLAB Device Blocks for Simulink
  wires:
  Data/1 -> UART Tx/1

== system microchip_mcb_pmsm_foc_qep/Serial Send/Subsystem/End ==
  Data : Inport
  Action Port : ActionPort  ActionPortLabel=elseif(u1 == 119)
  Mux : Mux  Inputs=2
  Start : Constant  Value=hex2dec('45')  OutDataTypeStr=uint8
  UART Tx : MCHP_Blockset/BUS UART/UART Tx  UART_REF=UART 0  ORDERING=None  AllOrNothing=off  SampleTime=-1  MCHP_MASTERLINK=microchip_mcb_pmsm_foc_qep/Configurations/Microchip Master  NSend_Input=off  UART_String=off  NSend_Output=off
      settings: SourceProductName=MPLAB Device Blocks for Simulink
  wires:
  Mux/1 -> UART Tx/1
  Data/1 -> Mux/1
  Start/1 -> Mux/2

== system microchip_mcb_pmsm_foc_qep/Serial Send/Subsystem/Start ==
  Data : Inport
  Action Port : ActionPort  ActionPortLabel=if(u1 == 0)
  End : Constant  Value=hex2dec('53')  OutDataTypeStr=uint8
  Mux : Mux  Inputs=2
  UART Tx : MCHP_Blockset/BUS UART/UART Tx  UART_REF=UART 0  ORDERING=None  AllOrNothing=off  SampleTime=-1  MCHP_MASTERLINK=microchip_mcb_pmsm_foc_qep/Configurations/Microchip Master  NSend_Input=off  UART_String=off  NSend_Output=off
      settings: SourceProductName=MPLAB Device Blocks for Simulink
  wires:
  Mux/1 -> UART Tx/1
  Data/1 -> Mux/2
  End/1 -> Mux/1

== system microchip_mcb_pmsm_foc_qep/Current Control/Closed Loop/OpenLoop/Mode Selector ==
  Enable : EnablePort
  1 sec : Constant  Value=1*PWM_frequency  OutDataTypeStr=uint32
  2 sec : Constant  Value=2*PWM_frequency  OutDataTypeStr=uint32
  Add1 : Sum  SaturateOnIntegerOverflow=on
  Constant : Constant  OutDataTypeStr=uint32
  Delay : Delay  DelayLength=1
  If : If  NumInputs=3  IfExpression=u1 < u2  ElseIfExpressions=u1 < u3
  If Action Subsystem : Subsystem  TreatAsAtomicUnit=on
  If Action Subsystem1 : Subsystem  TreatAsAtomicUnit=on
  If Action Subsystem2 : Subsystem  TreatAsAtomicUnit=on
  Merge : Merge  Inputs=3
  PositionOffsetEn : Outport
  wires:
  If Action Subsystem2/1(Out1) -> Merge/3
  Add1/1 -> If/1, Delay/1  "Count"
  1 sec/1 -> If/2
  2 sec/1 -> If/3
  If/1 -> If Action Subsystem/Action
  If/2 -> If Action Subsystem1/Action
  If/3 -> If Action Subsystem2/Action
  If Action Subsystem/1(Out1) -> Merge/1
  If Action Subsystem1/1(Out1) -> Merge/2
  Constant/1 -> Add1/1
  Delay/1 -> Add1/2
  Merge/1 -> PositionOffsetEn/1

== system microchip_mcb_pmsm_foc_qep/Current Control/Closed Loop/Subsystem/Current_Controllers ==
  Id : Inport
  Iq : Inport  Port=2
  Idq_Ref : Inport  Port=3
  DQ Limiter : mcbcontrolslib/DQ Limiter  Vmax=1
      settings: SourceProductBaseCode=MT
  Demux : Demux  Outputs=2
  Mux : Mux
  PI_Controller_Id : Subsystem
  PI_Controller_Iq : Subsystem
  Terminator : Terminator
  Vd_ref : Outport  VectorParamsAs1DForOutWhenUnconnected=off
  Vq_ref : Outport  Port=2  VectorParamsAs1DForOutWhenUnconnected=off
  Idq : Outport  Port=3  VectorParamsAs1DForOutWhenUnconnected=off
  wires:
  Iq/1 -> Mux/4, PI_Controller_Iq/2(I_fb)  "Iq_fb"
  PI_Controller_Id/1(V_ref) -> DQ Limiter/1
  Id/1 -> PI_Controller_Id/2(I_fb), Mux/2  "Id_fb"
  Demux/1 -> PI_Controller_Id/1(I_ref), Mux/1  "Id_Ref"
  Demux/2 -> Mux/3, PI_Controller_Iq/1(I_ref)  "Iq_Ref"
  DQ Limiter/1 -> Vd_ref/1
  DQ Limiter/2 -> Vq_ref/1
  PI_Controller_Iq/1(V_ref) -> DQ Limiter/2
  DQ Limiter/3 -> Terminator/1
  Idq_Ref/1 -> Demux/1
  Mux/1 -> Idq/1

== system microchip_mcb_pmsm_foc_qep/Current Control/Input Scaling/Calculate Position and Speed/Position Offset ==
  Iab : Inport
  Enable : EnablePort
  Offset : Outport
  wires:
  Iab/1 -> Offset/1

== system microchip_mcb_pmsm_foc_qep/Inverter and Motor - Plant Model/Plant Model/Inverter and Motor (sim)/Inverter ==
  Duty_abc : Inport
  Average-Value Inverter : mcbplantlib/Average-Value Inverter
  Constant2 : Constant  Value=inverter.V_dc  OutDataTypeStr=single  SampleTime=-1
  Data Type Conversion1 : DataTypeConversion  OutDataTypeStr=single  RndMeth=Simplest
  Rate Transition3 : RateTransition  Deterministic=off  OutPortSampleTime=Ts_inverter
  Vabc : Outport  VectorParamsAs1DForOutWhenUnconnected=off
  wires:
  Constant2/1 -> Average-Value Inverter/2
  Data Type Conversion1/1 -> Rate Transition3/1
  Duty_abc/1 -> Data Type Conversion1/1
  Average-Value Inverter/1 -> Vabc/1
  Rate Transition3/1 -> Average-Value Inverter/1

== system microchip_mcb_pmsm_foc_qep/Inverter and Motor - Plant Model/Plant Model/Inverter and Motor (sim)/Load_Profile (Torque) ==
  Data Type Conversion : DataTypeConversion  OutDataTypeStr=single
  IIR Filter : mcbcontrolslib/IIR Filter  VariantControl=Low Pass Filter  VariantSelect=Low-pass  Filter_constant=0.0001  advancedSettings=off  Ts=50e-6  cutOff_freq=0.31834
      settings: SourceProductBaseCode=MT
  T_load : Step  Time=4  Before=0.05*pmsm.T_rated  After=0.3*pmsm.T_rated  SampleTime=Ts_simulink
  Load_Trq : Outport  VectorParamsAs1DForOutWhenUnconnected=off
  wires:
  Data Type Conversion/1 -> IIR Filter/1
  IIR Filter/1 -> Load_Trq/1
  T_load/1 -> Data Type Conversion/1

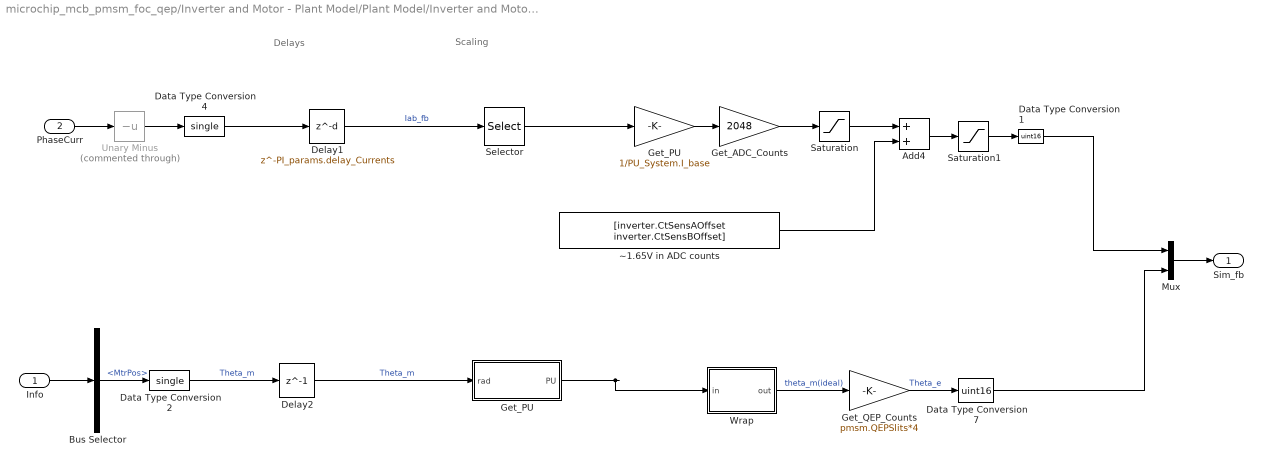
== system microchip_mcb_pmsm_foc_qep/Inverter and Motor - Plant Model/Plant Model/Inverter and Motor (sim)/Sensor_Measurements ==
  note: Scaling
  note: Delays
  Info : Inport
  PhaseCurr : Inport  Port=2
  Add4 : Sum  OutDataTypeStr=uint16
  Bus Selector : BusSelector  OutputSignals=MtrPos
  Data Type Conversion1 : DataTypeConversion  OutDataTypeStr=uint16
  Data Type Conversion2 : DataTypeConversion  OutDataTypeStr=single  RndMeth=Simplest
  Data Type Conversion4 : DataTypeConversion  OutDataTypeStr=single  RndMeth=Simplest
  Data Type Conversion7 : DataTypeConversion  OutDataTypeStr=uint16  RndMeth=Simplest
  Delay1 : Delay  DelayLength=PI_params.delay_Currents
  Delay2 : Delay  DelayLength=1
  Get_ADC_Counts : Gain  Gain=2048  RndMeth=Simplest  OutDataTypeStr=Inherit: Same as input
  Get_PU : Gain  Gain=1/PU_System.I_base  RndMeth=Simplest
  "Get_PU " : Subsystem
  Get_QEP_Counts : Gain  Gain=pmsm.QEPSlits*4  OutDataTypeStr=uint16  RndMeth=Simplest
  Mux : Mux  Inputs=2
  Saturation : Saturate  UpperLimit=2048  LowerLimit=-2048
  Saturation1 : Saturate  UpperLimit=4095  LowerLimit=0
  Selector : Selector  InputPortWidth=3  IndexOptions=Index vector (dialog)  Indices=[1 2]  OutputSizes=1
  Unary Minus : UnaryMinus  Commented=through
  Wrap : Subsystem
  ~1.65V in ADC counts : Constant  Value=[inverter.CtSensAOffset inverter.CtSensBOffset]  OutDataTypeStr=uint16  SampleTime=-1
  Sim_fb : Outport  VectorParamsAs1DForOutWhenUnconnected=off
  wires:
  Get_ADC_Counts/1 -> Saturation/1
  Saturation1/1 -> Data Type Conversion1/1
  Add4/1 -> Saturation1/1
  ~1.65V in ADC counts/1 -> Add4/2
  Delay1/1 -> Selector/1  "Iab_fb"
  Saturation/1 -> Add4/1
  Data Type Conversion4/1 -> Delay1/1
  PhaseCurr/1 -> Unary Minus/1
  Get_PU/1 -> Get_ADC_Counts/1
  Data Type Conversion1/1 -> Mux/1
  Selector/1 -> Get_PU/1
  Unary Minus/1 -> Data Type Conversion4/1
  Info/1 -> Bus Selector/1
  Data Type Conversion7/1 -> Mux/2
  "Get_PU "/1(PU) -> Wrap/1(in)
  Wrap/1(out) -> Get_QEP_Counts/1  "theta_m(ideal)"
  Delay2/1 -> "Get_PU "/1(rad)  "Theta_m"
  Get_QEP_Counts/1 -> Data Type Conversion7/1  "Theta_e"
  Data Type Conversion2/1 -> Delay2/1  "Theta_m"
  Bus Selector/1 -> Data Type Conversion2/1  "<MtrPos>"
  Mux/1 -> Sim_fb/1

== system microchip_mcb_pmsm_foc_qep/Serial Receive/CodeGen/Subsystem/unParse ==
  Data : Inport
  Bitwise Operator : simulink/Logic and Bit Operations/Bitwise Operator  logicop=AND  UseBitMask=on  BitMask=hex2dec('0001')  BitMaskRealWorld=Stored Integer
  Bitwise Operator1 : simulink/Logic and Bit Operations/Bitwise Operator  logicop=AND  UseBitMask=on  BitMask=hex2dec('00F0')  BitMaskRealWorld=Stored Integer
  Data Type Conversion3 : DataTypeConversion  OutDataTypeStr=boolean  RndMeth=Simplest
  Data Type Conversion4 : DataTypeConversion  OutDataTypeStr=uint16  RndMeth=Simplest
  Shift Arithmetic1 : ArithShift  BitShiftNumber=4
  Enable_PWM : Outport
  Debug_signals : Outport  Port=2
  wires:
  Bitwise Operator1/1 -> Shift Arithmetic1/1
  Data/1 -> Bitwise Operator/1, Bitwise Operator1/1
  Bitwise Operator/1 -> Data Type Conversion3/1
  Data Type Conversion4/1 -> Debug_signals/1
  Shift Arithmetic1/1 -> Data Type Conversion4/1
  Data Type Conversion3/1 -> Enable_PWM/1

== system microchip_mcb_pmsm_foc_qep/Serial Receive/CodeGen/Subsystem1/Triggered Subsystem ==
  In1 : Inport
  Enable : EnablePort
  Data out : Outport
  wires:
  In1/1 -> Data out/1

== system microchip_mcb_pmsm_foc_qep/Current Control/Closed Loop/OpenLoop/Mode Selector/If Action Subsystem ==
  Action Port : ActionPort  ActionPortLabel=if(u1 < u2)
  Constant1 : Constant  OutDataTypeStr=Inherit: Inherit via back propagation
  Counter Free-Running : simulink/Sources/Counter Free-Running  NumBits=12  tsamp=-1
  Data Store Write2 : DataStoreWrite  DataStoreName=EnPosOffset  IndexOptions=Index vector (dialog)  Indices=1  OutputSizes=1
  Gain : Gain  Gain=1/2^12  OutDataTypeStr=dataType  RndMeth=Simplest
  Out1 : Outport
  wires:
  Constant1/1 -> Data Store Write2/1
  Gain/1 -> Out1/1
  Counter Free-Running/1 -> Gain/1

== system microchip_mcb_pmsm_foc_qep/Current Control/Closed Loop/OpenLoop/Mode Selector/If Action Subsystem1 ==
  Action Port : ActionPort  ActionPortLabel=elseif(u1 < u3)
  Constant : Constant  Value=0  OutDataTypeStr=dataType
  Constant1 : Constant  OutDataTypeStr=Inherit: Inherit via back propagation
  Data Store Write2 : DataStoreWrite  DataStoreName=EnPosOffset  IndexOptions=Index vector (dialog)  Indices=1  OutputSizes=1
  Out1 : Outport
  wires:
  Constant1/1 -> Data Store Write2/1
  Constant/1 -> Out1/1
